simulink model "adaptive_cruise_control_student_version_2018a"  (R2019b)
settings: Solver=ode45  StartTime=0.0  StopTime=tend  MaxStep=0.01  RelTol=1e-12  AbsTol=1e-14  EnableMultiTasking=on
values from neighbouring files (symbols this model uses):
  a = 1/tau    [run_simulation.m]    (also in set_simulation_parameters.m = 0)
  dbar = 0*g*sin(theta)    [set_simulation_parameters.m]
  distance_far_away = 3000    [set_simulation_parameters.m]
  initial_cutoff_distance = 5    [set_simulation_parameters.m]
  is_cutoff_manoeuvre = false    [set_simulation_parameters.m]
  omega = 10    [set_simulation_parameters.m]
  q_0 = 80    [set_simulation_parameters.m]
  qdot_0 = 50    [set_simulation_parameters.m]
  qdot_ref = 100    [set_simulation_parameters.m]
  ql_0 = 100    [set_simulation_parameters.m]
  r = 10    [set_simulation_parameters.m]
  t_cutoff = 30    [set_simulation_parameters.m]
  vL = 80    [set_simulation_parameters.m]
  Vmax = 1000    [set_simulation_parameters.m]
libraries: simulink x5, dspsigops x1
settings Model: Creator=cnielsen  LastModifiedBy=batman
settings DataIOCC: LimitDataPoints=on  SaveFormat=Array  SaveOutput=off  DSMLogging=off  SaveTime=off  ReturnWorkspaceOutputs=off
settings OptimizationCC: ExpressionDepthLimit=2147483647  LifeSpan=inf
settings DebuggingCC: UnderspecifiedInitializationDetection=Classic  MergeDetectMultiDrivingBlocksExec=none  FcnCallInpInsideContextMsg=warning  StateNameClashWarn=warning  SFUnexpectedBacktrackingDiag=warning  SFNoUnconditionalDefaultTransitionDiag=warning  SFExecutionAtInitializationDiag=none  ArithmeticOperatorsInVariantConditions=warning
settings HardwareCC: ProdBitPerPointer=32  ProdBitPerSizeT=32  ProdBitPerPtrDiffT=32  ProdLargestAtomicFloat=None  ProdIntDivRoundTo=Undefined  ProdEndianess=Unspecified  ProdWordSize=32  ProdHWDeviceType=32-bit Generic
settings ModelReferenceCC: PropagateSignalLabelsOutOfModel=off
settings SFSimCC: SimUseLocalCustomCode=off  CustomCodeUndefinedFunction=UseInterfaceOnly
settings RTWCC: RTWUseLocalCustomCode=off
settings CodeAppCC: StateflowObjectComments=on
settings GRTTargetCC: TargetLangStandard=C89/C90 (ANSI)  GeneratePreprocessorConditionals=Disable all  CombineOutputUpdateFcns=off  GRTInterface=on
settings ConfigComp: CovMetricSettings=dw  CovHtmlReporting=on  CovSaveCumulativeToWorkspaceVar=on  CovSaveSingleToWorkspaceVar=on  CovExternalEMLEnable=off

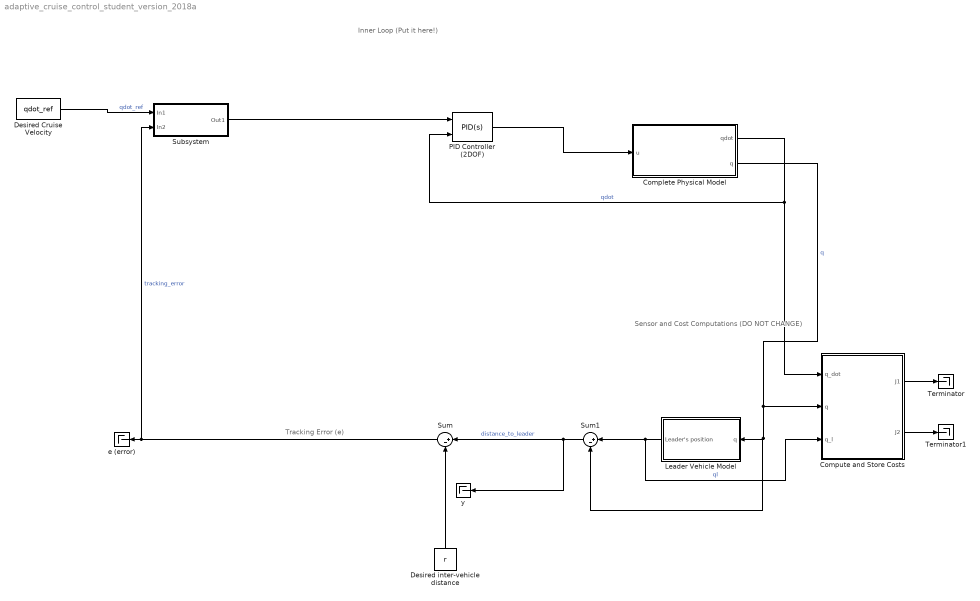
== system adaptive_cruise_control_student_version_2018a ==
  note: Tracking Error (e)
  note: Sensor and Cost Computations (DO NOT CHANGE)
  note: Inner Loop (Put it here!)
  Complete Physical Model : Subsystem
  Compute and Store Costs : Subsystem  AncestorBlock=HelpfulBlocks_R2018a/Compute and Store Costs
  Desired Cruise Velocity : Constant  Value=qdot_ref
  Desired inter-vehicle distance : Constant  Value=r
  Leader Vehicle Model : Subsystem  AncestorBlock=HelpfulBlocks_R2018a/Leader Vehicle Model
  PID Controller (2DOF) : simulink/Continuous/PID Controller (2DOF)  Controller=PID  Form=Parallel  TimeDomain=Continuous-time  SampleTime=-1  IntegratorMethod=Forward Euler  FilterMethod=Forward Euler  ControllerParametersSource=internal  P=409.92014787617  I=308.050705469526  D=-11.2474030949838  UseFilter=on  N=4  b=0.48830039062227  c=4.44911964658633  TunerSelectOption=Transfer Function Based (PID Tuner App)  InitialConditionSource=internal  InitialConditionForIntegrator=0  InitialConditionForFilter=0  DifferentiatorICPrevScaledInput=0  ExternalReset=none  TrackingMode=off  Kt=1  LimitOutput=on  UpperSaturationLimit=1000  LowerSaturationLimit=-1000  LinearizeAsGain=on  AntiWindupMode=back-calculation  Kb=1  POutMin=[]  POutMax=[]  IOutMin=[]  IOutMax=[]  DOutMin=[]  DOutMax=[]  NOutMin=[]  NOutMax=[]  bOutMin=[]  bOutMax=[]  cOutMin=[]  cOutMax=[]  SumOutMin=[]  SumOutMax=[]  SaturationOutMin=[]  SaturationOutMax=[]  PParamMin=[]  PParamMax=[]  IParamMin=[]  IParamMax=[]  DParamMin=[]  DParamMax=[]  NParamMin=[]  NParamMax=[]  bParamMin=[]  bParamMax=[]  cParamMin=[]  cParamMax=[]  KbParamMin=[]  KbParamMax=[]  KtParamMin=[]  KtParamMax=[]  KbOutMin=[]  KbOutMax=[]  KtOutMin=[]  KtOutMax=[]  IntegratorOutMin=[]  IntegratorOutMax=[]  FilterOutMin=[]  FilterOutMax=[]  SumI1OutMin=[]  SumI1OutMax=[]  SumI2OutMin=[]  SumI2OutMax=[]  SumI3OutMin=[]  SumI3OutMax=[]  SumI4OutMin=[]  SumI4OutMax=[]  SumDOutMin=[]  SumDOutMax=[]  Sum1OutMin=[]  Sum1OutMax=[]  Sum2OutMin=[]  Sum2OutMax=[]  Sum3OutMin=[]  Sum3OutMax=[]  DifferentiatorOutMin=[]  DifferentiatorOutMax=[]  FilterDiffOutCoefMin=[]  FilterDiffOutCoefMax=[]  ReciprocalOutMin=[]  ReciprocalOutMax=[]  SumDenOutMin=[]  SumDenOutMax=[]  SumNumOutMin=[]  SumNumOutMax=[]  DivideOutMin=[]  DivideOutMax=[]  IntegratorContinuousStateAttributes=''  IntegratorStateMustResolveToSignalObject=off  IntegratorRTWStateStorageClass=Auto  FilterContinuousStateAttributes=''  FilterStateMustResolveToSignalObject=off  FilterRTWStateStorageClass=Auto  ParallelPVariant=InternalParameters  IdealPVariant=Disabled  IVariant=InternalParameters  DVariant=InternalParameters  bVariant=InternalParameters  cVariant=InternalParameters  IntegratorVariant=Continuous  SatVariant=Enabled  AWVariant=BackCalculation  PCopyVariant=Disabled  TRVariant=Disabled  FdbkBlocksVariant=Forward  IdealPFdbkVariant=Disabled  SatFdbkVariant=Disabled  DerivativeFilterVariant=ContFilter  NVariant=InternalParameters  NCopyVariant=Disabled  FilterICVariant=InternalICsFilter  IntegratorICVariant=InternalICs  ExternalResetVariant=Disabled  TRSumVariant=Passthrough  SumFdbkVariant=Disabled  SumVariant=Sum_PID
  Subsystem : Subsystem
  Sum : Sum  Inputs=|+-
  Sum1 : Sum  Inputs=|+-
  Terminator : Terminator
  Terminator1 : Terminator
  e (error) : Terminator
  y : Terminator
  wires:
  Leader Vehicle Model/1(Leader's position) -> Sum1/1, Compute and Store Costs/3(q_l)  "ql"
  Compute and Store Costs/1(J1) -> Terminator/1
  Compute and Store Costs/2(J2) -> Terminator1/1
  Sum1/1 -> y/1, Sum/1  "distance_to_leader"
  Sum/1 -> Subsystem/2(In2), e (error)/1  "tracking_error"
  Desired inter-vehicle distance/1 -> Sum/2
  Complete Physical Model/1(qdot) -> Compute and Store Costs/1(q_dot), PID Controller (2DOF)/2  "qdot"
  Complete Physical Model/2(q) -> Compute and Store Costs/2(q), Sum1/2, Leader Vehicle Model/1(q)  "q"
  PID Controller (2DOF)/1 -> Complete Physical Model/1(u)
  Desired Cruise Velocity/1 -> Subsystem/1(In1)  "qdot_ref"
  Subsystem/1(Out1) -> PID Controller (2DOF)/1

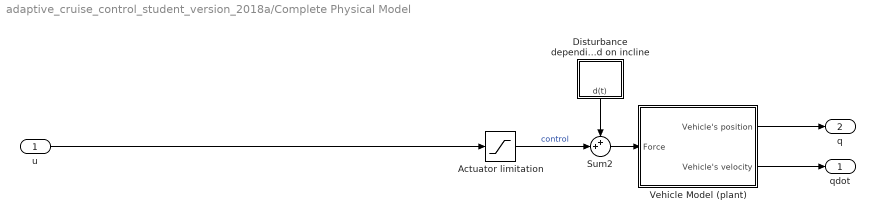
== system adaptive_cruise_control_student_version_2018a/Complete Physical Model ==
  u : Inport
  Actuator limitation : Saturate  UpperLimit=Vmax  LowerLimit=-Vmax
  Disturbance depending road on incline : Subsystem
  Sum2 : Sum  Inputs=++|
  Vehicle Model (plant) : Subsystem
  qdot : Outport
  q : Outport  Port=2
  wires:
  Disturbance depending road on incline/1(d(t)) -> Sum2/1
  Actuator limitation/1 -> Sum2/2  "control"
  Sum2/1 -> Vehicle Model (plant)/1(Force)
  Vehicle Model (plant)/1(Vehicle's position) -> q/1
  Vehicle Model (plant)/2(Vehicle's velocity) -> qdot/1
  u/1 -> Actuator limitation/1

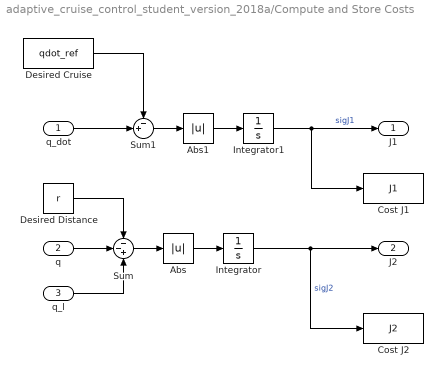
== system adaptive_cruise_control_student_version_2018a/Compute and Store Costs ==
  q_dot : Inport
  q : Inport  Port=2
  q_l : Inport  Port=3
  Abs : Abs
  Abs1 : Abs
  Cost J1 : ToWorkspace  VariableName=J1  SampleTime=-1
      settings: MaxDataPoints=1
  Cost J2 : ToWorkspace  VariableName=J2  SampleTime=-1
      settings: MaxDataPoints=1
  Desired Cruise : Constant  Value=qdot_ref
  Desired Distance : Constant  Value=r
  Integrator : Integrator
  Integrator1 : Integrator
  Sum : Sum  Inputs=--+
  Sum1 : Sum  Inputs=-+|
  J1 : Outport  VectorParamsAs1DForOutWhenUnconnected=off
  J2 : Outport  Port=2  VectorParamsAs1DForOutWhenUnconnected=off
  wires:
  q_l/1 -> Sum/3
  q/1 -> Sum/2
  Desired Distance/1 -> Sum/1
  Sum/1 -> Abs/1
  Abs/1 -> Integrator/1
  Integrator/1 -> Cost J2/1, J2/1  "sigJ2"
  q_dot/1 -> Sum1/2
  Desired Cruise/1 -> Sum1/1
  Sum1/1 -> Abs1/1
  Integrator1/1 -> Cost J1/1, J1/1  "sigJ1"
  Abs1/1 -> Integrator1/1

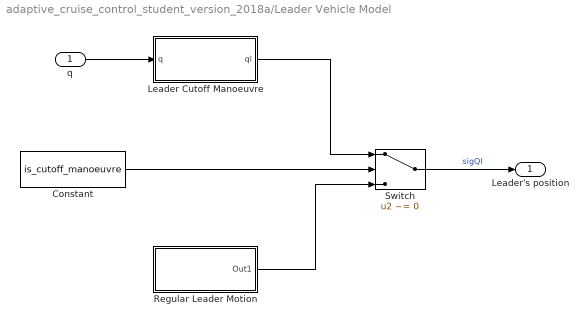
== system adaptive_cruise_control_student_version_2018a/Leader Vehicle Model ==
  q : Inport
  Constant : Constant  Value=is_cutoff_manoeuvre
  Leader Cutoff Manoeuvre : Subsystem
  Regular Leader Motion : Subsystem
  Switch : Switch  Criteria=u2 ~= 0
  Leader's position : Outport  VectorParamsAs1DForOutWhenUnconnected=off
  wires:
  Constant/1 -> Switch/2
  Switch/1 -> Leader's position/1  "sigQl"
  q/1 -> Leader Cutoff Manoeuvre/1(q)
  Leader Cutoff Manoeuvre/1(ql) -> Switch/1
  Regular Leader Motion/1(Out1) -> Switch/3

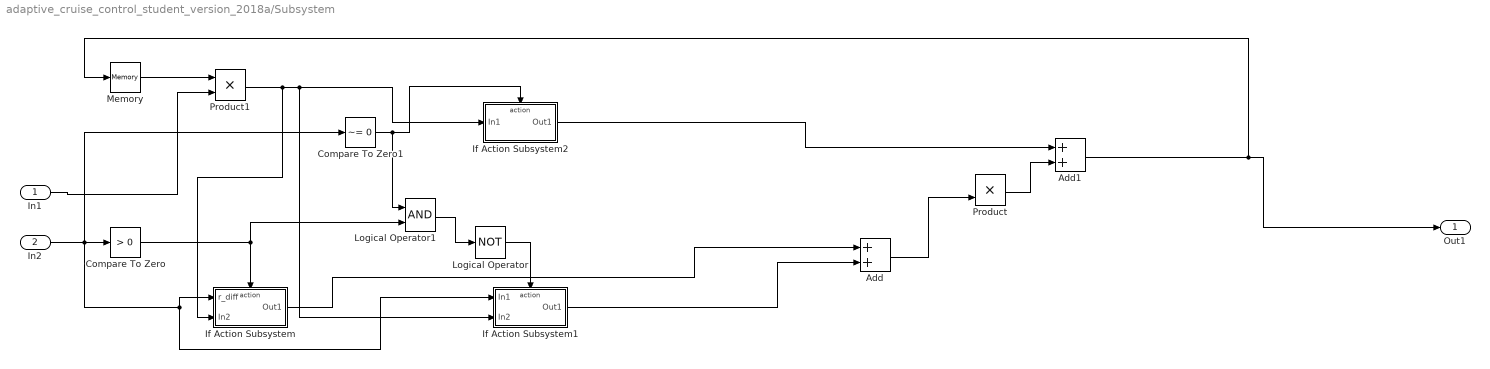
== system adaptive_cruise_control_student_version_2018a/Subsystem ==
  In1 : Inport
  In2 : Inport  Port=2
  Add : Sum
  Add1 : Sum
  Compare To Zero : simulink/Logic and Bit Operations/Compare To Zero  relop=>  OutDataTypeStr=boolean
  Compare To Zero1 : simulink/Logic and Bit Operations/Compare To Zero  relop=~=  OutDataTypeStr=boolean
  If Action Subsystem : Subsystem  TreatAsAtomicUnit=on
  If Action Subsystem1 : Subsystem  TreatAsAtomicUnit=on
  If Action Subsystem2 : Subsystem  TreatAsAtomicUnit=on
  Logical Operator : Logic  Operator=NOT  AllPortsSameDT=off  OutDataTypeStr=boolean
  Logical Operator1 : Logic  AllPortsSameDT=off  OutDataTypeStr=boolean
  Memory : Memory  InitialCondition=1  InheritSampleTime=on
  Product : Product
  Product1 : Product
  Out1 : Outport
  wires:
  In2/1 -> If Action Subsystem1/1(In1), If Action Subsystem/1(r_diff), Compare To Zero1/1, Compare To Zero/1
  Compare To Zero/1 -> If Action Subsystem/Action, Logical Operator1/2
  Logical Operator/1 -> If Action Subsystem1/Action
  In1/1 -> Product1/2
  If Action Subsystem/1(Out1) -> Add/1
  If Action Subsystem1/1(Out1) -> Add/2
  Add/1 -> Product/2
  Compare To Zero1/1 -> Logical Operator1/1, If Action Subsystem2/Action
  Logical Operator1/1 -> Logical Operator/1
  Product/1 -> Add1/2
  If Action Subsystem2/1(Out1) -> Add1/1
  Add1/1 -> Memory/1, Out1/1
  Memory/1 -> Product1/1
  Product1/1 -> If Action Subsystem/2(In2), If Action Subsystem1/2(In2), If Action Subsystem2/1(In1)

== system adaptive_cruise_control_student_version_2018a/Complete Physical Model/Disturbance depending road on incline ==
  Step : Step  Time=0  After=dbar  SampleTime=0
  d(t) : Outport  VectorParamsAs1DForOutWhenUnconnected=off
  wires:
  Step/1 -> d(t)/1

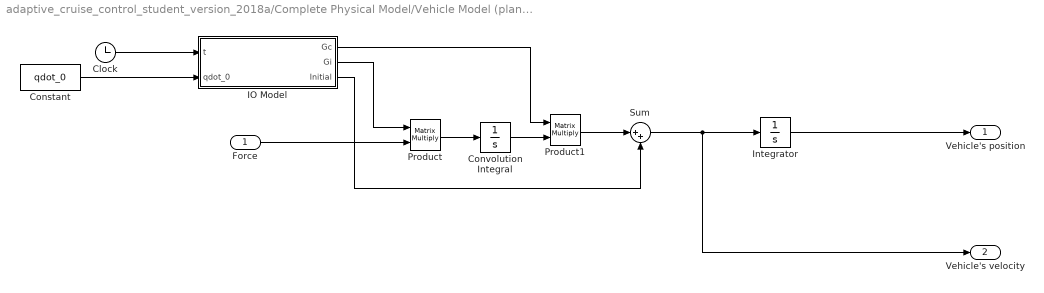
== system adaptive_cruise_control_student_version_2018a/Complete Physical Model/Vehicle Model (plant) ==
  Force : Inport
  Clock : Clock
  Constant : Constant  Value=qdot_0
  Convolution Integral : Integrator
  IO Model : MATLAB Function  TreatAsAtomicUnit=on  RTWFcnName=UnknownPlant
      settings: RTWFileNameOpts=Use function name
  Integrator : Integrator  InitialCondition=q_0
  Product : Product  Multiplication=Matrix(*)
  Product1 : Product  Multiplication=Matrix(*)
  Sum : Sum  Inputs=|++
  Vehicle's position : Outport  VectorParamsAs1DForOutWhenUnconnected=off
  Vehicle's velocity : Outport  Port=2  VectorParamsAs1DForOutWhenUnconnected=off
  wires:
  Integrator/1 -> Vehicle's position/1
  Clock/1 -> IO Model/1(t)
  Product/1 -> Convolution Integral/1
  Convolution Integral/1 -> Product1/2
  IO Model/1(Gc) -> Product1/1
  Force/1 -> Product/2
  IO Model/2(Gi) -> Product/1
  Constant/1 -> IO Model/2(qdot_0)
  Product1/1 -> Sum/1
  Sum/1 -> Vehicle's velocity/1, Integrator/1
  IO Model/3(Initial) -> Sum/2

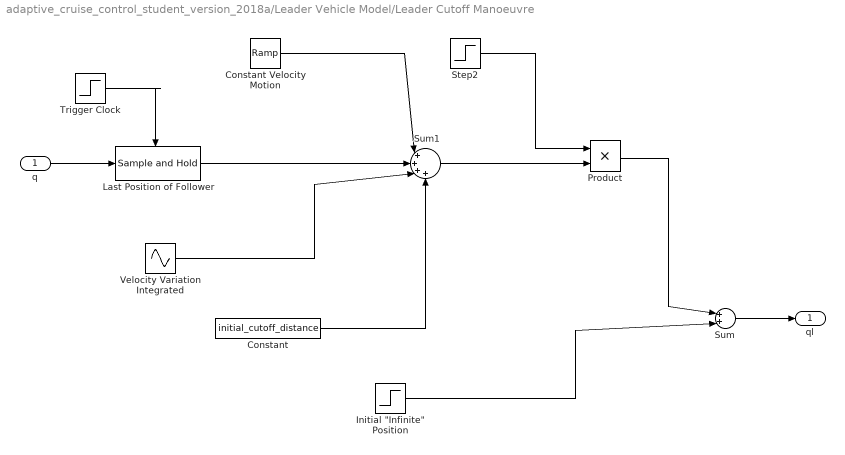
== system adaptive_cruise_control_student_version_2018a/Leader Vehicle Model/Leader Cutoff Manoeuvre ==
  q : Inport
  Constant : Constant  Value=initial_cutoff_distance
  Constant Velocity Motion : simulink/Sources/Ramp  slope=vL  start=t_cutoff  InitialOutput=0
  "Initial \"Infinite\" Position" : Step  Time=t_cutoff  Before=distance_far_away  After=0  SampleTime=0
  Last Position of Follower : dspsigops/Sample and Hold  trig=Rising edge  initCond=0  latchinput=off
  Product : Product
  Step2 : Step  Time=t_cutoff  SampleTime=0
  Sum : Sum  Inputs=|++|
  Sum1 : Sum  Inputs=|++++
  Trigger Clock : Step  Time=t_cutoff  Before=-1  SampleTime=0
  Velocity Variation Integrated : Sin  Amplitude=a/omega  Frequency=omega  SampleTime=0
  ql : Outport
  wires:
  q/1 -> Last Position of Follower/1
  Trigger Clock/1 -> Last Position of Follower/Trigger
  Sum/1 -> ql/1
  "Initial \"Infinite\" Position"/1 -> Sum/2
  Sum1/1 -> Product/2
  Step2/1 -> Product/1
  Product/1 -> Sum/1
  Last Position of Follower/1 -> Sum1/2
  Velocity Variation Integrated/1 -> Sum1/3
  Constant/1 -> Sum1/4
  Constant Velocity Motion/1 -> Sum1/1

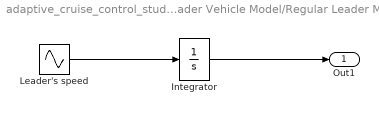
== system adaptive_cruise_control_student_version_2018a/Leader Vehicle Model/Regular Leader Motion ==
  Integrator : Integrator  InitialCondition=ql_0
  Leader's speed : Sin  Amplitude=a  Bias=vL  Frequency=omega  SampleTime=0
  Out1 : Outport
  wires:
  Leader's speed/1 -> Integrator/1
  Integrator/1 -> Out1/1

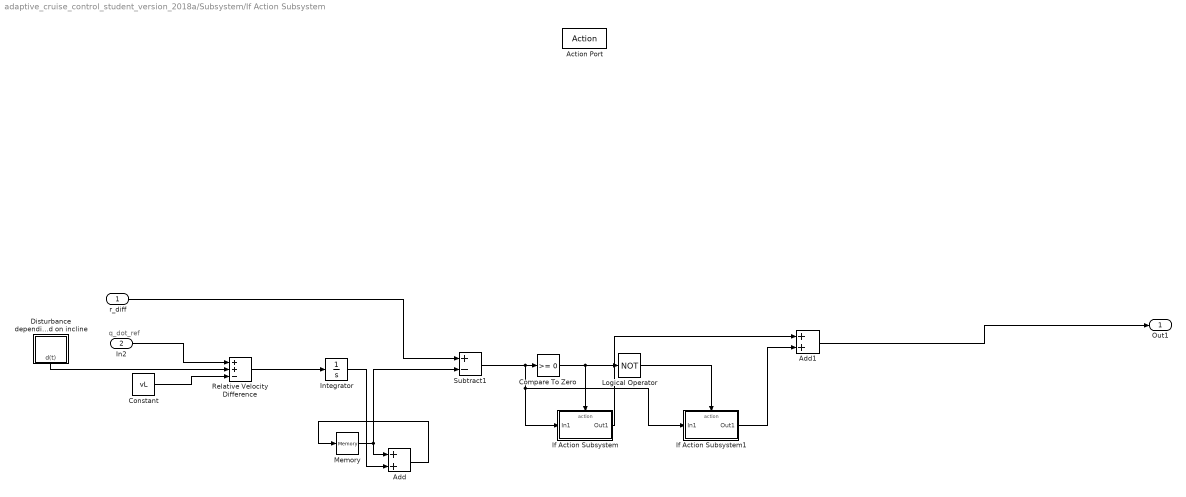
== system adaptive_cruise_control_student_version_2018a/Subsystem/If Action Subsystem ==
  note: q_dot_ref
  r_diff : Inport
  In2 : Inport  Port=2
  Action Port : ActionPort
  Add : Sum
  Add1 : Sum
  Compare To Zero : simulink/Logic and Bit Operations/Compare To Zero  relop=>=  OutDataTypeStr=boolean
  Constant : Constant  Value=vL
  Disturbance depending road on incline : Subsystem
  If Action Subsystem : Subsystem  TreatAsAtomicUnit=on
  If Action Subsystem1 : Subsystem  TreatAsAtomicUnit=on
  Integrator : Integrator
  Logical Operator : Logic  Operator=NOT  AllPortsSameDT=off  OutDataTypeStr=boolean
  Memory : Memory  InheritSampleTime=on
  "Relative Velocity Difference " : Sum  Inputs=++-
  Subtract1 : Sum  Inputs=+-
  Out1 : Outport
  wires:
  In2/1 -> "Relative Velocity Difference "/1
  Constant/1 -> "Relative Velocity Difference "/3
  Disturbance depending road on incline/1(d(t)) -> "Relative Velocity Difference "/2
  "Relative Velocity Difference "/1 -> Integrator/1
  Integrator/1 -> Add/2
  Memory/1 -> Add/1, Subtract1/2
  Add/1 -> Memory/1
  r_diff/1 -> Subtract1/1
  Subtract1/1 -> If Action Subsystem1/1(In1), If Action Subsystem/1(In1), Compare To Zero/1
  Compare To Zero/1 -> If Action Subsystem/Action, Logical Operator/1
  Logical Operator/1 -> If Action Subsystem1/Action
  If Action Subsystem1/1(Out1) -> Add1/2
  If Action Subsystem/1(Out1) -> Add1/1
  Add1/1 -> Out1/1

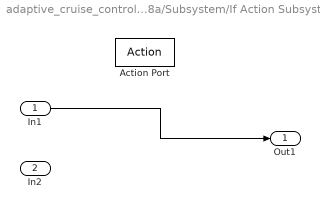
== system adaptive_cruise_control_student_version_2018a/Subsystem/If Action Subsystem1 ==
  In1 : Inport
  In2 : Inport  Port=2
  Action Port : ActionPort
  Out1 : Outport
  wires:
  In1/1 -> Out1/1

== system adaptive_cruise_control_student_version_2018a/Subsystem/If Action Subsystem2 ==
  In1 : Inport
  Action Port : ActionPort
  Out1 : Outport
  wires:
  In1/1 -> Out1/1

== system adaptive_cruise_control_student_version_2018a/Subsystem/If Action Subsystem/Disturbance depending road on incline ==
  Step : Step  Time=0  After=dbar  SampleTime=0
  d(t) : Outport  VectorParamsAs1DForOutWhenUnconnected=off
  wires:
  Step/1 -> d(t)/1

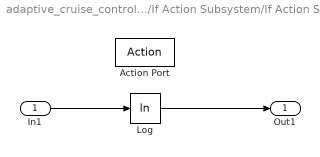
== system adaptive_cruise_control_student_version_2018a/Subsystem/If Action Subsystem/If Action Subsystem ==
  In1 : Inport
  Action Port : ActionPort
  Log : Math  Operator=log  SaturateOnIntegerOverflow=on
  Out1 : Outport
  wires:
  In1/1 -> Log/1
  Log/1 -> Out1/1

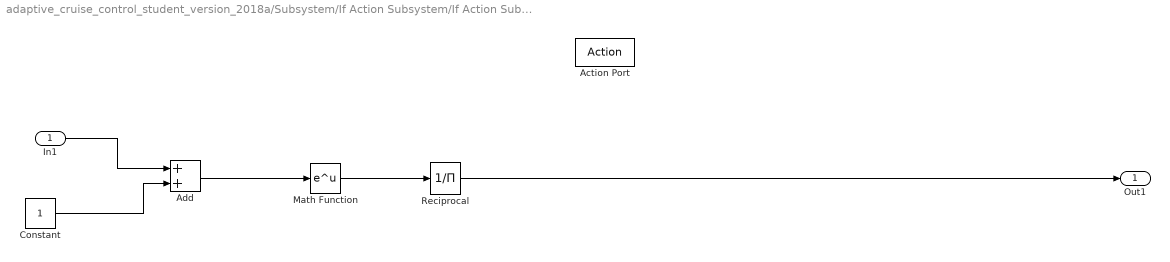
== system adaptive_cruise_control_student_version_2018a/Subsystem/If Action Subsystem/If Action Subsystem1 ==
  In1 : Inport
  Action Port : ActionPort
  Add : Sum
  Constant : Constant
  Math Function : Math  SignedPower=off  SaturateOnIntegerOverflow=on
  Reciprocal : Product  Inputs=/
  Out1 : Outport
  wires:
  In1/1 -> Add/1
  Constant/1 -> Add/2
  Add/1 -> Math Function/1
  Math Function/1 -> Reciprocal/1
  Reciprocal/1 -> Out1/1

== matlab function adaptive_cruise_control_student_version_2018a/Complete Physical Model/Vehicle Model (plant)/IO Model ==
  data: t input; Gc output; Gi output; qdot_0 input; Initial output
function [Gc, Gi, Initial] = InternalPlant(t, qdot_0)
[Gc, Gi, Initial] = UnknownPlant(t, qdot_0);
